simulink model "phaser"  (R2025b)
settings: Solver=FixedStepDiscrete  StartTime=0.0  StopTime=inf  RelTol=1e-3
undefined symbols (not defined in the file): Depth_rt, Dry_rt, Feedback_rt, Freq_rt, Repeats_rt, Time_rt, Wet_rt
settings Model: Creator=linogarciamorales  LastModifiedBy=linogarciamorales
settings OptimizationCC: EnhancedBackFolding=on  PassReuseOutputArgsAs=Individual arguments  ZeroExternalMemoryAtStartup=off  ZeroInternalMemoryAtStartup=off  OptimizeBlockOrder=speed  DifferentSizesBufferReuse=on  OptimizationCustomize=off  EfficientTunableParamExpr=on
settings DebuggingCC: ParameterTunabilityLossMsg=error
settings SFSimCC: MATLABDynamicMemAlloc=off
settings RTWCC: SystemTargetFile=ert.tlc  GenCodeOnly=on  TemplateMakefile=ert_default_tmf  Description=Embedded Coder
settings CodeAppCC: ForceParamTrailComments=on  IgnoreCustomStorageClasses=off  OperatorAnnotations=on  SimulinkDataObjDesc=on  SFDataObjDesc=on  InsertBlockDesc=on
settings ERTTargetCC: InlinedParameterPlacement=Hierarchical  ERTCustomFileTemplate=example_file_process.tlc  TargetLangStandard=C99 (ISO)  GenerateSampleERTMain=on  SupportNonInlinedSFcns=on

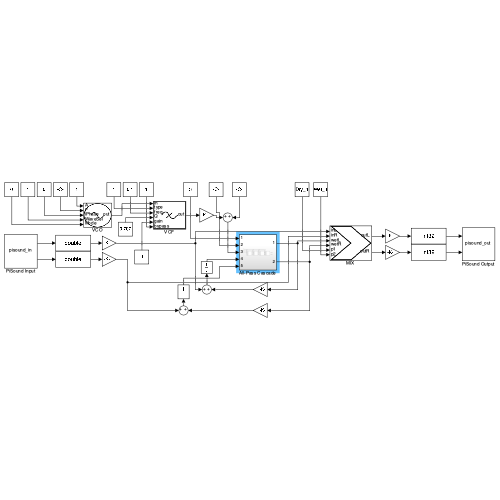
[thumbnail: Simulink's stored preview of the top-level diagram]
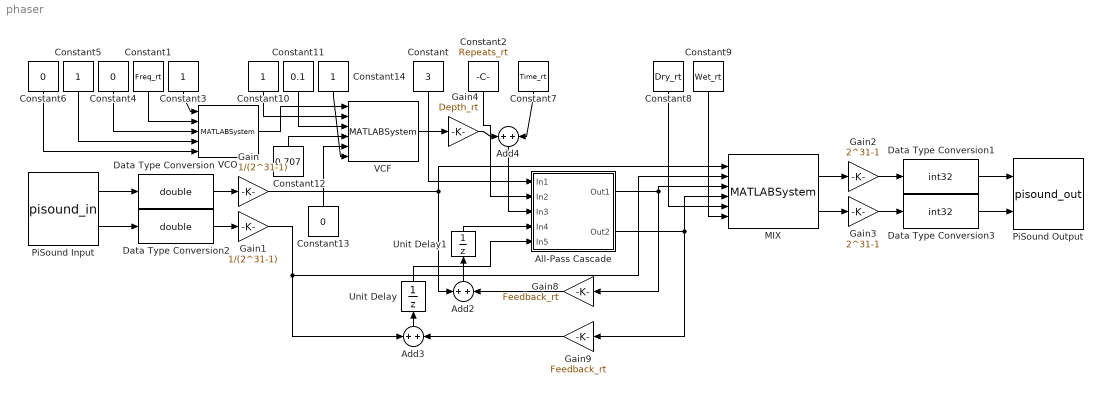
== system phaser ==
  Add2 : Sum  OutDataTypeStr=double  AccumDataTypeStr=double
  Add3 : Sum  OutDataTypeStr=double  AccumDataTypeStr=double
  Add4 : Sum  OutDataTypeStr=double  AccumDataTypeStr=double
  All-Pass Cascade : Subsystem
  Constant : Constant  Value=3  OutDataTypeStr=uint8
  Constant1 : Constant  Value=Freq_rt  OutDataTypeStr=double
  Constant10 : Constant  OutDataTypeStr=uint8
  Constant11 : Constant  Value=0.1  OutDataTypeStr=double
  Constant12 : Constant  Value=0.707  OutDataTypeStr=double
  Constant13 : Constant  Value=0  OutDataTypeStr=double
  Constant14 : Constant  OutDataTypeStr=double
  Constant2 : Constant  Value=Repeats_rt  OutDataTypeStr=double
  Constant3 : Constant  OutDataTypeStr=double
  Constant4 : Constant  Value=0  OutDataTypeStr=double
  Constant5 : Constant  OutDataTypeStr=uint8
  Constant6 : Constant  Value=0  OutDataTypeStr=uint8
  Constant7 : Constant  Value=Time_rt  OutDataTypeStr=double
  Constant8 : Constant  Value=Dry_rt  OutDataTypeStr=double
  Constant9 : Constant  Value=Wet_rt  OutDataTypeStr=double
  Data Type Conversion : DataTypeConversion  OutDataTypeStr=double  SaturateOnIntegerOverflow=off  RndMeth=Floor
  Data Type Conversion1 : DataTypeConversion  OutDataTypeStr=int32  SaturateOnIntegerOverflow=off  RndMeth=Floor
  Data Type Conversion2 : DataTypeConversion  OutDataTypeStr=double  SaturateOnIntegerOverflow=off  RndMeth=Floor
  Data Type Conversion3 : DataTypeConversion  OutDataTypeStr=int32  SaturateOnIntegerOverflow=off  RndMeth=Floor
  Gain : Gain  Gain=1/(2^31-1)
  Gain1 : Gain  Gain=1/(2^31-1)
  Gain2 : Gain  Gain=2^31-1
  Gain3 : Gain  Gain=2^31-1
  Gain4 : Gain  Gain=Depth_rt
  Gain8 : Gain  Gain=Feedback_rt  OutDataTypeStr=double
  Gain9 : Gain  Gain=Feedback_rt  OutDataTypeStr=double
  MIX : MATLABSystem  System=mix_sys  N=128  Fs=48000  Mode=uint8(2)  SmoothTime=0.01  IndepInDB=false  SimulateUsing=Code generation
      mask Type: mix_sys
  PiSound Input : S-Function  FunctionName=pisound_in  Parameters=48000, 128, 0  SFunctionDeploymentMode=off  EnableBusSupport=off
  PiSound Output : S-Function  FunctionName=pisound_out  Parameters=48000, 128, 0  SFunctionDeploymentMode=off  EnableBusSupport=off
  Unit Delay : UnitDelay  SampleTime=-1  HasFrameUpgradeWarning=on
  Unit Delay1 : UnitDelay  SampleTime=-1  HasFrameUpgradeWarning=on
  VCF : MATLABSystem  System=vcf_mono_sys  N=128  Fs=48000  SimulateUsing=Code generation
      mask Type: vcf_mono_sys
  VCO : MATLABSystem  System=vco_mono_sys  N=128  Fs=48000  OutMaxL=4096  InFixL=1024  SimulateUsing=Code generation
      mask Type: vco_mono_sys
  wires:
  PiSound Input/2 -> Data Type Conversion2/1
  Data Type Conversion1/1 -> PiSound Output/1
  Data Type Conversion3/1 -> PiSound Output/2
  Gain2/1 -> Data Type Conversion1/1
  Gain3/1 -> Data Type Conversion3/1
  Data Type Conversion/1 -> Gain/1
  Data Type Conversion2/1 -> Gain1/1
  Gain/1 -> MIX/1, Add2/1
  Gain1/1 -> Add3/1, MIX/2
  MIX/1 -> Gain2/1
  MIX/2 -> Gain3/1
  Constant1/1 -> VCO/2
  Constant3/1 -> VCO/1
  Constant4/1 -> VCO/3
  Constant5/1 -> VCO/4
  Constant6/1 -> VCO/5
  Add2/1 -> Unit Delay1/1
  Gain8/1 -> Add2/2
  Add3/1 -> Unit Delay/1
  Gain9/1 -> Add3/2
  Constant8/1 -> MIX/5
  VCO/1 -> VCF/1
  Constant7/1 -> Add4/2
  Constant9/1 -> MIX/6
  Gain4/1 -> Add4/1
  VCF/1 -> Gain4/1
  Constant10/1 -> VCF/2
  Constant11/1 -> VCF/3
  Constant12/1 -> VCF/4
  Constant13/1 -> VCF/5
  Constant14/1 -> VCF/6
  All-Pass Cascade/2(Out2) -> MIX/4, Gain9/1
  All-Pass Cascade/1(Out1) -> MIX/3, Gain8/1
  Constant/1 -> All-Pass Cascade/1(In1)
  Constant2/1 -> All-Pass Cascade/2(In2)
  Add4/1 -> All-Pass Cascade/3(In3)
  Unit Delay1/1 -> All-Pass Cascade/4(In4)
  Unit Delay/1 -> All-Pass Cascade/5(In5)
  PiSound Input/1 -> Data Type Conversion/1

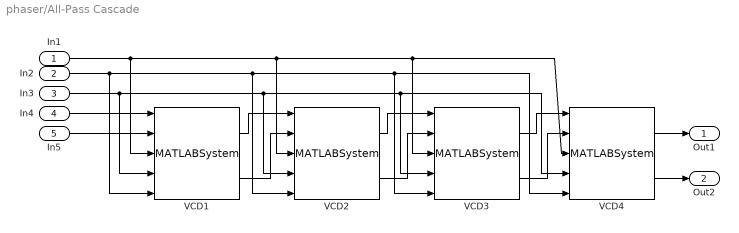
== system phaser/All-Pass Cascade ==
  In1 : Inport
  In2 : Inport  Port=2
  In3 : Inport  Port=3
  In4 : Inport  Port=4
  In5 : Inport  Port=5
  VCD{1..4} (4 alike) : MATLABSystem  System=vcd_sys  N=128  Fs=48000  MaxDelay=2  Mode=uint8(1)  Delay=0.1  g=0.5  SimulateUsing=Code generation
      mask Type: vcd_sys
  Out1 : Outport
  Out2 : Outport  Port=2
  wires:
  In4/1 -> VCD1/1
  In1/1 -> VCD1/3, VCD3/3, VCD4/3, VCD2/3
  In3/1 -> VCD1/4, VCD2/4, VCD4/4, VCD3/4
  In5/1 -> VCD1/2
  In2/1 -> VCD3/5, VCD4/5, VCD2/5, VCD1/5
  VCD1/1 -> VCD2/1
  VCD1/2 -> VCD2/2
  VCD2/1 -> VCD3/1
  VCD2/2 -> VCD3/2
  VCD4/1 -> Out1/1
  VCD4/2 -> Out2/1
  VCD3/1 -> VCD4/1
  VCD3/2 -> VCD4/2
